simulink model "PI_Controller0"  (R2020a)
settings: Solver=ode45  StartTime=0.0  StopTime=120  RelTol=1e-3
undefined symbols (not defined in the file): Ki, Kp, Ts
settings Model: DataDictionary=CruiseCtrl_data.sldd  Creator=NIKITA  LastModifiedBy=NIKITA
settings DataIOCC: SaveOutput=off  SaveTime=off

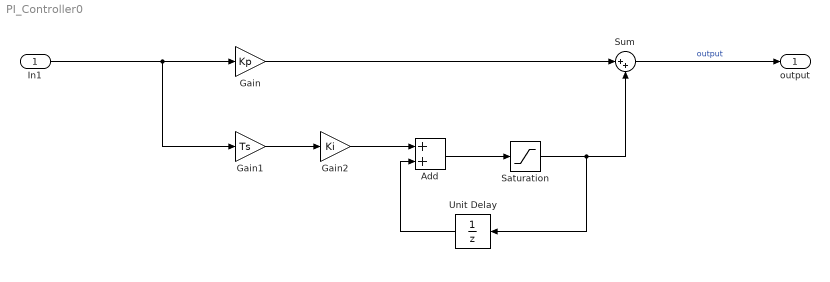
== system PI_Controller0 ==
  In1 : Inport  OutDataTypeStr=double  PortDimensions=1  SampleTime=0
  Add : Sum
  Gain : Gain  Gain=Kp
  Gain1 : Gain  Gain=Ts
  Gain2 : Gain  Gain=Ki
  Saturation : Saturate  UpperLimit=1  LowerLimit=-1
  Sum : Sum  Inputs=|++
  Unit Delay : UnitDelay  SampleTime=-1  HasFrameUpgradeWarning=on
  output : Outport  OutDataTypeStr=double  PortDimensions=1  SampleTime=0
  wires:
  Gain/1 -> Sum/1
  Saturation/1 -> Unit Delay/1, Sum/2
  Gain2/1 -> Add/1
  Add/1 -> Saturation/1
  Unit Delay/1 -> Add/2
  Gain1/1 -> Gain2/1
  In1/1 -> Gain/1, Gain1/1
  Sum/1 -> output/1  "output"
